simulink model "motor_drive_model"  (R2022a)
settings: Solver=VariableStepAuto  StartTime=0.0  StopTime=0.1  RelTol=0.001
undefined symbols (not defined in the file): J, k, kE, kF, kM, L, Mnom, n, R, Unom
settings Model: Creator=clever0ne  LastModifiedBy=clever0ne
settings SolverCC: ZeroCrossAlgorithm=Adaptive
settings DataIOCC: SaveFormat=Array  ReturnWorkspaceOutputs=off
settings DebuggingCC: IgnoredZcDiagnostic=none

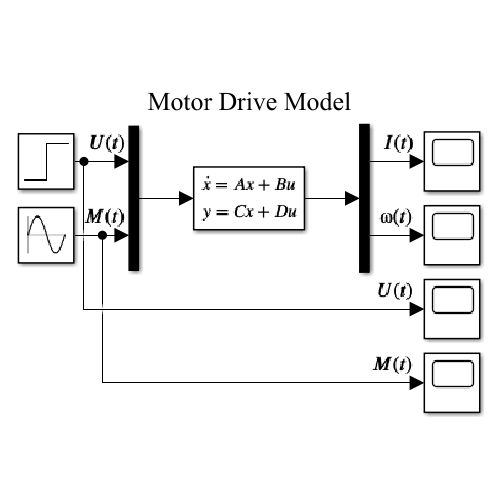
[thumbnail: Simulink's stored preview of the top-level diagram]
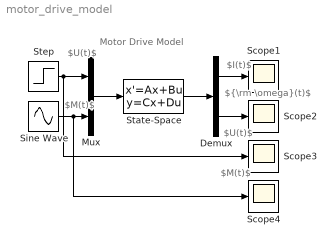
== system motor_drive_model ==
  note: $U(t)$
  note: Motor Drive Model
  note: $M(t)$
  note: $M(t)$
  note: $U(t)$
  note: $I(t)$
  note: ${\rm \omega}(t)$
  Demux : Demux  Outputs=2
  Mux : Mux  Inputs=2
  Scope{1..4} (4 alike) : Scope
  Sine Wave : Sin  Amplitude=0.3 * n * k * Mnom  Bias=-n * k * Mnom  Frequency=20 * pi  SampleTime=0
  State-Space : StateSpace  A=[-R/L, -k*kE/L; n*k*kM/J, -kF/J]  B=[1/L, 0; 0, 1/J]  C=eye(2)  D=zeros(2)  InitialCondition=0
  Step : Step  Time=0.0001  After=Unom  SampleTime=0
  wires:
  State-Space/1 -> Demux/1
  Demux/2 -> Scope2/1
  Demux/1 -> Scope1/1
  Step/1 -> Mux/1, Scope3/1
  Mux/1 -> State-Space/1
  Sine Wave/1 -> Scope4/1, Mux/2
